simulink model "exSim"  (R2019b)
settings: Solver=VariableStepAuto  StartTime=0.0  StopTime=300  RelTol=1e-3
settings Model: Creator=ovi  LastModifiedBy=ovi

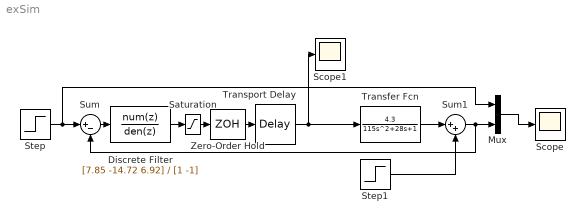
== system exSim ==
  Discrete Filter : DiscreteFilter  Numerator=[7.85 -14.72 6.92]  Denominator=[1 -1]  SampleTime=0.5
  Mux : Mux  Inputs=2
  Saturation : Saturate  UpperLimit=0.6  LowerLimit=0
  Scope : Scope
  Scope1 : Scope
  Step : Step  SampleTime=0
  Step1 : Step  After=0  SampleTime=0
  Sum : Sum  Inputs=|+-
  Sum1 : Sum  Inputs=|++
  Transfer Fcn : TransferFcn  Numerator=[4.3]  Denominator=[115 28 1]
  Transport Delay : TransportDelay  DelayTime=2.5
  Zero-Order Hold : ZeroOrderHold  SampleTime=0.5
  wires:
  Step/1 -> Mux/1, Sum/1
  Transport Delay/1 -> Scope1/1, Transfer Fcn/1
  Sum/1 -> Discrete Filter/1
  Zero-Order Hold/1 -> Transport Delay/1
  Transfer Fcn/1 -> Sum1/1
  Sum1/1 -> Mux/2, Sum/2
  Step1/1 -> Sum1/2
  Mux/1 -> Scope/1
  Discrete Filter/1 -> Saturation/1
  Saturation/1 -> Zero-Order Hold/1
